simulink model "Areodynamic_Coefficient"  (R2022a)
settings: Solver=VariableStepAuto  StartTime=0.0  StopTime=1  RelTol=1e-3
undefined symbols (not defined in the file): a1, ac, AeroCoeff, b1
libraries: aerolibconvert2 x4
(part 1 of 2)
settings Model: Creator=user  LastModifiedBy=user
settings SolverCC: AlgebraicLoopSolver=TrustRegion
settings DataIOCC: SaveOutput=off  SaveTime=off  ReturnWorkspaceOutputs=off
settings DebuggingCC: UnconnectedInputMsg=warning  UnconnectedOutputMsg=warning  UnconnectedLineMsg=warning  SFMachineParentedDataDiag=warning

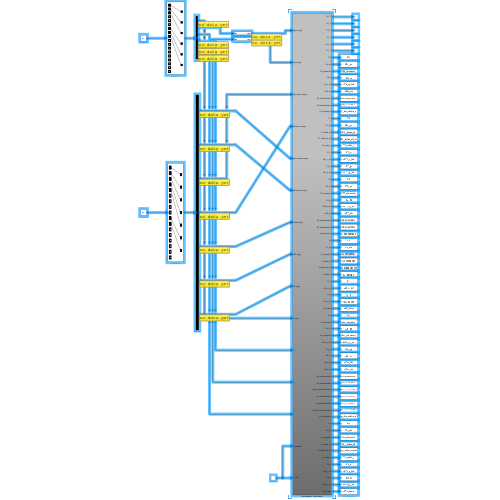
[thumbnail: Simulink's stored preview of the top-level diagram]
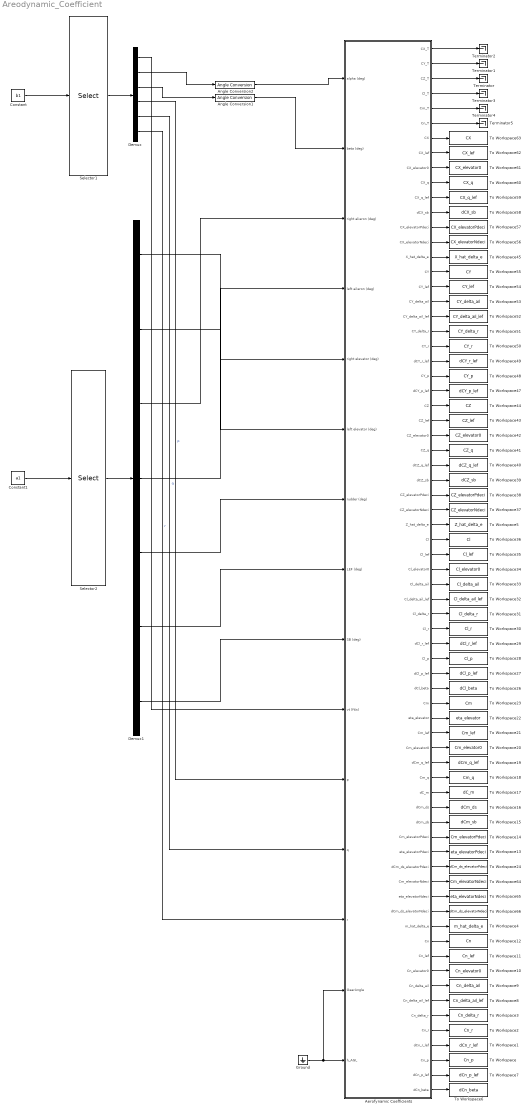
== system Areodynamic_Coefficient ==
  Aerofynamic Coefficients : Subsystem
  Angle Conversion1 : aerolibconvert2/Angle Conversion  IU=rad  OU=deg
  Angle Conversion2 : aerolibconvert2/Angle Conversion  IU=rad  OU=deg
  Constant : Constant  Value=b1
  Constant1 : Constant  Value=a1
  Demux : Demux  Outputs=6
  Demux1 : Demux  Outputs=7
  Ground : Ground
  Selector1 : Selector  InputPortWidth=18  IndexOptions=Index vector (dialog)  Indices=[1:3,7:9]  OutputSizes=3
  Selector2 : Selector  InputPortWidth=17  IndexOptions=Index vector (dialog)  Indices=[1:5 10 11]  OutputSizes=3
  Terminator{,1..5} (6 alike) : Terminator
  To Workspace : ToWorkspace  VariableName=Cn_p  SampleTime=-1
  To Workspace1 : ToWorkspace  VariableName=dCn_r_lef  SampleTime=-1
  To Workspace10 : ToWorkspace  VariableName=Cn_elevator0  SampleTime=-1
  To Workspace11 : ToWorkspace  VariableName=Cn_lef  SampleTime=-1
  To Workspace12 : ToWorkspace  VariableName=Cn  SampleTime=-1
  To Workspace13 : ToWorkspace  VariableName=eta_elevatorPdeci  SampleTime=-1
  To Workspace14 : ToWorkspace  VariableName=Cm_elevatorPdeci  SampleTime=-1
  To Workspace15 : ToWorkspace  VariableName=dCm_sb  SampleTime=-1
  To Workspace16 : ToWorkspace  VariableName=dCm_ds  SampleTime=-1
  To Workspace17 : ToWorkspace  VariableName=dC_m  SampleTime=-1
  To Workspace18 : ToWorkspace  VariableName=Cm_q  SampleTime=-1
  To Workspace19 : ToWorkspace  VariableName=dCm_q_lef  SampleTime=-1
  To Workspace2 : ToWorkspace  VariableName=Cn_r  SampleTime=-1
  To Workspace20 : ToWorkspace  VariableName=Cm_elevator0  SampleTime=-1
  To Workspace21 : ToWorkspace  VariableName=Cm_lef  SampleTime=-1
  To Workspace22 : ToWorkspace  VariableName=eta_elevator  SampleTime=-1
  To Workspace23 : ToWorkspace  VariableName=Cm  SampleTime=-1
  To Workspace24 : ToWorkspace  VariableName=dCm_ds_elevatorPdeci  SampleTime=-1
  To Workspace26 : ToWorkspace  VariableName=dCl_beta  SampleTime=-1
  To Workspace27 : ToWorkspace  VariableName=dCl_p_lef  SampleTime=-1
  To Workspace28 : ToWorkspace  VariableName=Cl_p  SampleTime=-1
  To Workspace29 : ToWorkspace  VariableName=dCl_r_lef  SampleTime=-1
  To Workspace3 : ToWorkspace  VariableName=Cn_delta_r  SampleTime=-1
  To Workspace30 : ToWorkspace  VariableName=Cl_r  SampleTime=-1
  To Workspace31 : ToWorkspace  VariableName=Cl_delta_r  SampleTime=-1
  To Workspace32 : ToWorkspace  VariableName=Cl_delta_ail_lef  SampleTime=-1
  To Workspace33 : ToWorkspace  VariableName=Cl_delta_ail  SampleTime=-1
  To Workspace34 : ToWorkspace  VariableName=Cl_elevator0  SampleTime=-1
  To Workspace35 : ToWorkspace  VariableName=Cl_lef  SampleTime=-1
  To Workspace36 : ToWorkspace  VariableName=Cl  SampleTime=-1
  To Workspace37 : ToWorkspace  VariableName=CZ_elevatorNdeci  SampleTime=-1
  To Workspace38 : ToWorkspace  VariableName=CZ_elevatorPdeci  SampleTime=-1
  To Workspace39 : ToWorkspace  VariableName=dCZ_sb  SampleTime=-1
  To Workspace4 : ToWorkspace  VariableName=m_hat_delta_e  SampleTime=-1
  To Workspace40 : ToWorkspace  VariableName=dCZ_q_lef  SampleTime=-1
  To Workspace41 : ToWorkspace  VariableName=CZ_q  SampleTime=-1
  To Workspace42 : ToWorkspace  VariableName=CZ_elevator0  SampleTime=-1
  To Workspace43 : ToWorkspace  VariableName=CZ_lef  SampleTime=-1
  To Workspace44 : ToWorkspace  VariableName=CZ  SampleTime=-1
  To Workspace45 : ToWorkspace  VariableName=X_hat_delta_e  SampleTime=-1
  To Workspace47 : ToWorkspace  VariableName=dCY_p_lef  SampleTime=-1
  To Workspace48 : ToWorkspace  VariableName=CY_p  SampleTime=-1
  To Workspace49 : ToWorkspace  VariableName=dCY_r_lef  SampleTime=-1
  To Workspace5 : ToWorkspace  VariableName=Z_hat_delta_e  SampleTime=-1
  To Workspace50 : ToWorkspace  VariableName=CY_r  SampleTime=-1
  To Workspace51 : ToWorkspace  VariableName=CY_delta_r  SampleTime=-1
  To Workspace52 : ToWorkspace  VariableName=CY_delta_ail_lef  SampleTime=-1
  To Workspace53 : ToWorkspace  VariableName=CY_delta_ail  SampleTime=-1
  To Workspace54 : ToWorkspace  VariableName=CY_lef  SampleTime=-1
  To Workspace55 : ToWorkspace  VariableName=CY  SampleTime=-1
  To Workspace56 : ToWorkspace  VariableName=CX_elevatorNdeci  SampleTime=-1
  To Workspace57 : ToWorkspace  VariableName=CX_elevatorPdeci  SampleTime=-1
  To Workspace58 : ToWorkspace  VariableName=dCX_sb  SampleTime=-1
  To Workspace59 : ToWorkspace  VariableName=CX_q_lef  SampleTime=-1
  To Workspace6 : ToWorkspace  VariableName=dCn_beta  SampleTime=-1
  To Workspace60 : ToWorkspace  VariableName=CX_q  SampleTime=-1
  To Workspace61 : ToWorkspace  VariableName=CX_elevator0  SampleTime=-1
  To Workspace62 : ToWorkspace  VariableName=CX_lef  SampleTime=-1
  To Workspace63 : ToWorkspace  VariableName=CX  SampleTime=-1
  To Workspace64 : ToWorkspace  VariableName=Cm_elevatorNdeci  SampleTime=-1
  To Workspace65 : ToWorkspace  VariableName=eta_elevatorNdeci  SampleTime=-1
  To Workspace66 : ToWorkspace  VariableName=dCm_ds_elevatorNdeci  SampleTime=-1
  To Workspace7 : ToWorkspace  VariableName=dCn_p_lef  SampleTime=-1
  To Workspace8 : ToWorkspace  VariableName=Cn_delta_ail_lef  SampleTime=-1
  To Workspace9 : ToWorkspace  VariableName=Cn_delta_ail  SampleTime=-1
  wires:
  Ground/1 -> Aerofynamic Coefficients/14(GearAngle), Aerofynamic Coefficients/15(h_AGL)
  Aerofynamic Coefficients/3(CZ_T) -> Terminator/1
  Aerofynamic Coefficients/2(CY_T) -> Terminator1/1
  Aerofynamic Coefficients/1(CX_T) -> Terminator2/1
  Aerofynamic Coefficients/4(Cl_T) -> Terminator3/1
  Aerofynamic Coefficients/5(Cm_T) -> Terminator4/1
  Aerofynamic Coefficients/6(Cn_T) -> Terminator5/1
  Aerofynamic Coefficients/69(Cn_p) -> To Workspace/1
  Angle Conversion1/1 -> Aerofynamic Coefficients/2(beta (deg))
  Angle Conversion2/1 -> Aerofynamic Coefficients/1(alpha (deg))
  Demux/2 -> Angle Conversion2/1
  Selector1/1 -> Demux/1
  Demux/3 -> Angle Conversion1/1
  Demux/1 -> Aerofynamic Coefficients/10(vt (ft/s))
  Constant1/1 -> Selector2/1
  Selector2/1 -> Demux1/1
  Demux1/1 -> Aerofynamic Coefficients/5(right elevator (deg))
  Demux1/2 -> Aerofynamic Coefficients/6(left elevator (deg))
  Demux1/3 -> Aerofynamic Coefficients/3(right alieron (deg))
  Demux1/4 -> Aerofynamic Coefficients/4(left aileron (deg))
  Demux1/5 -> Aerofynamic Coefficients/7(rudder (deg))
  Demux1/6 -> Aerofynamic Coefficients/8(LEF (deg))
  Demux1/7 -> Aerofynamic Coefficients/9(SB (deg))
  Aerofynamic Coefficients/68(dCn_r_lef) -> To Workspace1/1
  Aerofynamic Coefficients/67(Cn_r) -> To Workspace2/1
  Aerofynamic Coefficients/66(Cn_delta_r) -> To Workspace3/1
  Aerofynamic Coefficients/71(dCn_beta) -> To Workspace6/1
  Aerofynamic Coefficients/70(dCn_p_lef) -> To Workspace7/1
  Aerofynamic Coefficients/65(Cn_delta_ail_lef) -> To Workspace8/1
  Aerofynamic Coefficients/64(Cn_delta_ail) -> To Workspace9/1
  Aerofynamic Coefficients/63(Cn_elevator0) -> To Workspace10/1
  Aerofynamic Coefficients/62(Cn_lef) -> To Workspace11/1
  Aerofynamic Coefficients/61(Cn) -> To Workspace12/1
  Aerofynamic Coefficients/55(eta_elevatorPdeci) -> To Workspace13/1
  Aerofynamic Coefficients/54(Cm_elevatorPdeci) -> To Workspace14/1
  Aerofynamic Coefficients/53(dCm_sb) -> To Workspace15/1
  Aerofynamic Coefficients/52(dCm_ds) -> To Workspace16/1
  Aerofynamic Coefficients/51(dC_m) -> To Workspace17/1
  Aerofynamic Coefficients/50(Cm_q) -> To Workspace18/1
  Aerofynamic Coefficients/49(dCm_q_lef) -> To Workspace19/1
  Aerofynamic Coefficients/48(Cm_elevator0) -> To Workspace20/1
  Aerofynamic Coefficients/47(Cm_lef) -> To Workspace21/1
  Aerofynamic Coefficients/46(eta_elevator) -> To Workspace22/1
  Aerofynamic Coefficients/45(Cm) -> To Workspace23/1
  Aerofynamic Coefficients/44(dCl_beta) -> To Workspace26/1
  Aerofynamic Coefficients/43(dCl_p_lef) -> To Workspace27/1
  Aerofynamic Coefficients/42(Cl_p) -> To Workspace28/1
  Aerofynamic Coefficients/41(dCl_r_lef) -> To Workspace29/1
  Aerofynamic Coefficients/40(Cl_r) -> To Workspace30/1
  Aerofynamic Coefficients/39(Cl_delta_r) -> To Workspace31/1
  Aerofynamic Coefficients/38(Cl_delta_ail_lef) -> To Workspace32/1
  Aerofynamic Coefficients/37(Cl_delta_ail) -> To Workspace33/1
  Aerofynamic Coefficients/36(Cl_elevator0) -> To Workspace34/1
  Aerofynamic Coefficients/35(Cl_lef) -> To Workspace35/1
  Aerofynamic Coefficients/34(Cl) -> To Workspace36/1
  Aerofynamic Coefficients/32(CZ_elevatorNdeci) -> To Workspace37/1
  Aerofynamic Coefficients/31(CZ_elevatorPdeci) -> To Workspace38/1
  Aerofynamic Coefficients/30(dCZ_sb) -> To Workspace39/1
  Aerofynamic Coefficients/29(dCZ_q_lef) -> To Workspace40/1
  Aerofynamic Coefficients/28(CZ_q) -> To Workspace41/1
  Aerofynamic Coefficients/27(CZ_elevator0) -> To Workspace42/1
  Aerofynamic Coefficients/26(CZ_lef) -> To Workspace43/1
  Aerofynamic Coefficients/25(CZ) -> To Workspace44/1
  Aerofynamic Coefficients/24(dCY_p_lef) -> To Workspace47/1
  Aerofynamic Coefficients/23(CY_p) -> To Workspace48/1
  Aerofynamic Coefficients/22(dCY_r_lef) -> To Workspace49/1
  Aerofynamic Coefficients/21(CY_r) -> To Workspace50/1
  Aerofynamic Coefficients/20(CY_delta_r) -> To Workspace51/1
  Aerofynamic Coefficients/19(CY_delta_ail_lef) -> To Workspace52/1
  Aerofynamic Coefficients/18(CY_delta_ail) -> To Workspace53/1
  Aerofynamic Coefficients/17(CY_lef) -> To Workspace54/1
  Aerofynamic Coefficients/16(CY) -> To Workspace55/1
  Aerofynamic Coefficients/14(CX_elevatorNdeci) -> To Workspace56/1
  Aerofynamic Coefficients/13(CX_elevatorPdeci) -> To Workspace57/1
  Aerofynamic Coefficients/12(dCX_sb) -> To Workspace58/1
  Aerofynamic Coefficients/11(CX_q_lef) -> To Workspace59/1
  Aerofynamic Coefficients/10(CX_q) -> To Workspace60/1
  Aerofynamic Coefficients/9(CX_elevator0) -> To Workspace61/1
  Aerofynamic Coefficients/8(CX_lef) -> To Workspace62/1
  Aerofynamic Coefficients/7(CX) -> To Workspace63/1
  Aerofynamic Coefficients/56(dCm_ds_elevatorPdeci) -> To Workspace24/1
  Aerofynamic Coefficients/57(Cm_elevatorNdeci) -> To Workspace64/1
  Aerofynamic Coefficients/58(eta_elevatorNdeci) -> To Workspace65/1
  Aerofynamic Coefficients/59(dCm_ds_elevatorNdeci) -> To Workspace66/1
  Aerofynamic Coefficients/60(m_hat_delta_e) -> To Workspace4/1
  Aerofynamic Coefficients/33(Z_hat_delta_e) -> To Workspace5/1
  Aerofynamic Coefficients/15(X_hat_delta_e) -> To Workspace45/1
  Constant/1 -> Selector1/1
  Demux/6 -> Aerofynamic Coefficients/13(r)  "r"
  Demux/5 -> Aerofynamic Coefficients/12(q)  "q"
  Demux/4 -> Aerofynamic Coefficients/11(p)  "p"

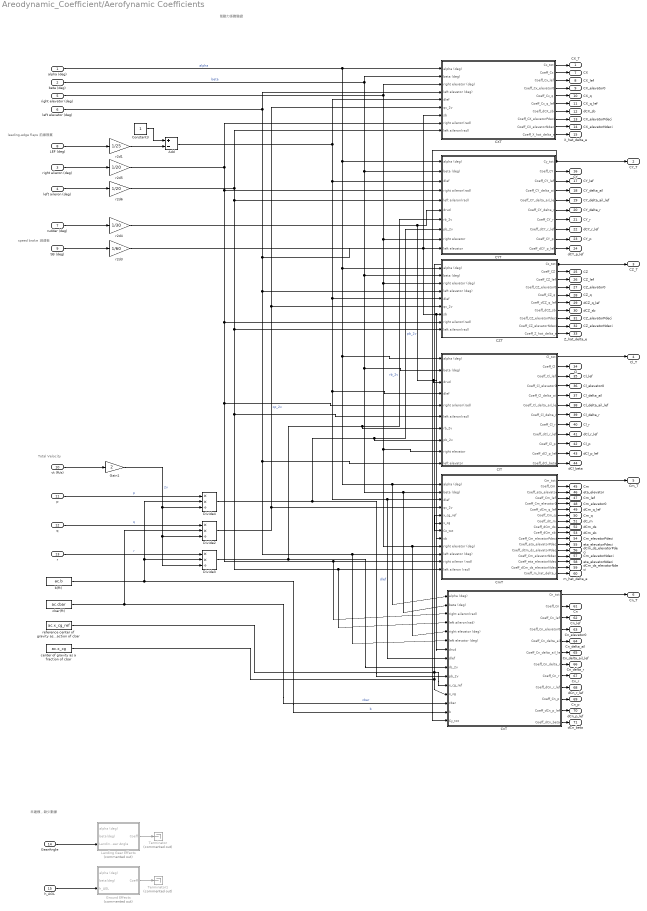
== system Areodynamic_Coefficient/Aerofynamic Coefficients ==
  note: 氣動力係數驗證
  note: Total Velocity
  note: 未建模，缺少數據
  note: speed brake
      | 減速板
  note: leading-edge flaps
      | 前緣襟翼
  alpha (deg) : Inport
  beta (deg) : Inport  Port=2
  right alieron (deg) : Inport  Port=3
  left aileron (deg) : Inport  Port=4
  right elevator (deg) : Inport  Port=5
  left elevator (deg) : Inport  Port=6
  rudder (deg) : Inport  Port=7
  LEF (deg) : Inport  Port=8
  SB (deg) : Inport  Port=9
  vt (ft/s) : Inport  Port=10
  p : Inport  Port=11
  q : Inport  Port=12
  r : Inport  Port=13
  GearAngle : Inport  Port=14
  h_AGL : Inport  Port=15
  Add : Sum  Inputs=+-
  CXT : Subsystem
  CYT : Subsystem
  CZT : Subsystem
  ClT : Subsystem
  CmT : Subsystem
  CnT : Subsystem
  Constant3 : Constant
  Divide2 : Product  Inputs=**/
  Divide3 : Product  Inputs=**/
  Divide4 : Product  Inputs=**/
  Gain1 : Gain  Gain=2
  Ground Effects : Subsystem  Commented=on
  Landing Gear Effects : Subsystem  Commented=on
  Terminator : Terminator  Commented=on
  Terminator1 : Terminator  Commented=on
  b(ft) : Constant  Value=ac.b
  cbar(ft) : Constant  Value=ac.cbar
  center of gravity as a fraction of cbar : Constant  Value=ac.x_cg
  r2d1 : Gain  Gain=1/25  SaturateOnIntegerOverflow=on  OutDataTypeStr=Inherit: Same as input  ParamDataTypeStr=Inherit: Same as input
  r2d3 : Gain  Gain=1/60  SaturateOnIntegerOverflow=on  OutDataTypeStr=Inherit: Same as input  ParamDataTypeStr=Inherit: Same as input
  r2d4 : Gain  Gain=1/30  SaturateOnIntegerOverflow=on  OutDataTypeStr=Inherit: Same as input  ParamDataTypeStr=Inherit: Same as input
  r2d5 : Gain  Gain=1/20  SaturateOnIntegerOverflow=on  OutDataTypeStr=Inherit: Same as input  ParamDataTypeStr=Inherit: Same as input
  r2d6 : Gain  Gain=1/20  SaturateOnIntegerOverflow=on  OutDataTypeStr=Inherit: Same as input  ParamDataTypeStr=Inherit: Same as input
  reference center of gravity as a fraction of cbar : Constant  Value=ac.x_cg_ref
  CX_T : Outport  VectorParamsAs1DForOutWhenUnconnected=off
  CY_T : Outport  Port=2  VectorParamsAs1DForOutWhenUnconnected=off
  CZ_T : Outport  Port=3  VectorParamsAs1DForOutWhenUnconnected=off
  Cl_T : Outport  Port=4  VectorParamsAs1DForOutWhenUnconnected=off
  Cm_T : Outport  Port=5  VectorParamsAs1DForOutWhenUnconnected=off
  Cn_T : Outport  Port=6  VectorParamsAs1DForOutWhenUnconnected=off
  CX : Outport  Port=7  VectorParamsAs1DForOutWhenUnconnected=off
  CX_lef : Outport  Port=8  VectorParamsAs1DForOutWhenUnconnected=off
  CX_elevator0 : Outport  Port=9  VectorParamsAs1DForOutWhenUnconnected=off
  CX_q : Outport  Port=10  VectorParamsAs1DForOutWhenUnconnected=off
  CX_q_lef : Outport  Port=11  VectorParamsAs1DForOutWhenUnconnected=off
  dCX_sb : Outport  Port=12  VectorParamsAs1DForOutWhenUnconnected=off
  CX_elevatorPdeci : Outport  Port=13  VectorParamsAs1DForOutWhenUnconnected=off
  CX_elevatorNdeci : Outport  Port=14  VectorParamsAs1DForOutWhenUnconnected=off
  X_hat_delta_e : Outport  Port=15
  CY : Outport  Port=16
  CY_lef : Outport  Port=17
  CY_delta_ail : Outport  Port=18
  CY_delta_ail_lef : Outport  Port=19
  CY_delta_r : Outport  Port=20
  CY_r : Outport  Port=21
  dCY_r_lef : Outport  Port=22
  CY_p : Outport  Port=23
  dCY_p_lef : Outport  Port=24
  CZ : Outport  Port=25
  CZ_lef : Outport  Port=26
  CZ_elevator0 : Outport  Port=27
  CZ_q : Outport  Port=28
  dCZ_q_lef : Outport  Port=29
  dCZ_sb : Outport  Port=30
  CZ_elevatorPdeci : Outport  Port=31
  CZ_elevatorNdeci : Outport  Port=32
  Z_hat_delta_e : Outport  Port=33
  Cl : Outport  Port=34
  Cl_lef : Outport  Port=35
  Cl_elevator0 : Outport  Port=36
  Cl_delta_ail : Outport  Port=37
  Cl_delta_ail_lef : Outport  Port=38
  Cl_delta_r : Outport  Port=39
  Cl_r : Outport  Port=40
  dCl_r_lef : Outport  Port=41
  Cl_p : Outport  Port=42
  dCl_p_lef : Outport  Port=43
  dCl_beta : Outport  Port=44
  Cm : Outport  Port=45
  eta_elevator : Outport  Port=46
  Cm_lef : Outport  Port=47
  Cm_elevator0 : Outport  Port=48
  dCm_q_lef : Outport  Port=49
  Cm_q : Outport  Port=50
  dC_m : Outport  Port=51
  dCm_ds : Outport  Port=52
  dCm_sb : Outport  Port=53
  Cm_elevatorPdeci : Outport  Port=54
  eta_elevatorPdeci : Outport  Port=55
  dCm_ds_elevatorPdeci : Outport  Port=56
  Cm_elevatorNdeci : Outport  Port=57
  eta_elevatorNdeci : Outport  Port=58
  dCm_ds_elevatorNdeci : Outport  Port=59
  m_hat_delta_e : Outport  Port=60
  Cn : Outport  Port=61
  Cn_lef : Outport  Port=62
  Cn_elevator0 : Outport  Port=63
  Cn_delta_ail : Outport  Port=64
  Cn_delta_ail_lef : Outport  Port=65
  Cn_delta_r : Outport  Port=66
  Cn_r : Outport  Port=67
  dCn_r_lef : Outport  Port=68
  Cn_p : Outport  Port=69
  dCn_p_lef : Outport  Port=70
  dCn_beta : Outport  Port=71
  wires:
  alpha (deg)/1 -> CnT/1(alpha (deg)), CmT/1(alpha (deg)), ClT/1(alpha (deg)), CZT/1(alpha (deg)), CYT/1(alpha (deg)), CXT/1(alpha (deg))  "alpha"
  beta (deg)/1 -> CnT/2(beta (deg)), CmT/2(beta (deg)), ClT/2(beta (deg)), CZT/2(beta (deg)), CYT/2(beta (deg)), CXT/2("beta (deg) ")  "beta"
  right elevator (deg)/1 -> CnT/5("right elevator (deg) "), CmT/9(right elevator (deg)), ClT/9(right elevator), CZT/3(right elevator (deg)), CYT/9(right elevator), CXT/3(right elevator (deg))
  vt (ft/s)/1 -> Gain1/1
  q/1 -> Divide2/1  "q"
  r/1 -> Divide3/1  "r"
  Divide2/1 -> CXT/6(qc_2v), CZT/6(qc_2v), CmT/4(qc_2v)  "qc_2v"
  Divide3/1 -> CYT/7(rb_2v), ClT/7(rb_2v), CnT/9(rb_2v)  "rb_2v"
  Divide4/1 -> CYT/8(pb_2v), ClT/8(pb_2v), CnT/10(pb_2v)  "pb_2v"
  b(ft)/1 -> CnT/14(b), Divide3/2, Divide4/2  "b"
  cbar(ft)/1 -> CnT/13(cbar), Divide2/2  "cbar"
  reference center of gravity as a fraction of cbar/1 -> CmT/5(x_cg_ref), CnT/11(x_cg_ref)
  center of gravity as a fraction of cbar/1 -> CmT/6(x_cg), CnT/12(x_cg)
  CZT/1(Cz_tot) -> CZ_T/1, CmT/7(Cz_tot)
  CYT/1(Cy_tot) -> CY_T/1, CnT/15(Cy_tot)
  CXT/1(Cx_tot) -> CX_T/1
  ClT/1(Cl_tot) -> Cl_T/1
  CmT/1(Cm_tot) -> Cm_T/1
  CnT/1(Cn_tot) -> Cn_T/1
  Add/1 -> CXT/5(dlef), CnT/8(dlef), CmT/3(dlef), ClT/4(dlef), CZT/5(dlef), CYT/3(dlef)  "dlef"
  rudder (deg)/1 -> r2d4/1
  SB (deg)/1 -> r2d3/1
  r2d1/1 -> Add/2
  Constant3/1 -> Add/1
  LEF (deg)/1 -> r2d1/1
  Gain1/1 -> Divide4/3, Divide3/3, Divide2/3  "2v"
  p/1 -> Divide4/1  "p"
  r2d3/1 -> CmT/8(sb), CZT/7(sb), CXT/7(sb)
  r2d4/1 -> CYT/6(drud), CnT/7(drud), ClT/3(drud)
  GearAngle/1 -> Landing Gear Effects/3(Landing Gear Angle)
  h_AGL/1 -> Ground Effects/3(h_AGL)
  Landing Gear Effects/1(Coeff) -> Terminator/1
  Ground Effects/1(Coeff) -> Terminator1/1
  left elevator (deg)/1 -> CnT/6(left elevator (deg)), CmT/10(left elevator (deg)), ClT/10(left elevator), CZT/4(left elevator (deg)), CYT/10(left elevator), CXT/4(left elevator (deg))
  right alieron (deg)/1 -> r2d5/1
  left aileron (deg)/1 -> r2d6/1
  r2d5/1 -> CnT/3(right aileron(rad)), CmT/11(right aileron (rad)), ClT/5(right aileron(rad)), CZT/8(right aileron(rad)), CYT/4(right aileron(rad)), CXT/8(right aileron(rad))
  r2d6/1 -> CXT/9(left aileron(rad)), CnT/4(left aileron(rad)), CmT/12(left aileron (rad)), ClT/6(left aileron(rad)), CZT/9(left aileron(rad)), CYT/5(left aileron(rad))
  CnT/10(Coeff_Cn_p) -> Cn_p/1
  CXT/2(Coeff_Cx) -> CX/1
  CXT/3(Coeff_Cx_lef) -> CX_lef/1
  CXT/4(Coeff_Cx_elevator0) -> CX_elevator0/1
  CXT/5(Coeff_Cx_q) -> CX_q/1
  CXT/6(Coeff_Cx_q_lef) -> CX_q_lef/1
  CXT/7(Coeff_dCX_sb) -> dCX_sb/1
  CXT/8(Coeff_CX_elevatorPdeci) -> CX_elevatorPdeci/1
  CXT/9(Coeff_CX_elevatorNdeci) -> CX_elevatorNdeci/1
  CYT/2(Coeff_CY) -> CY/1
  CYT/3(Coeff_CY_lef) -> CY_lef/1
  CYT/4(Coeff_CY_delta_ail) -> CY_delta_ail/1
  CYT/5(Coeff_CY_delta_ail_lef) -> CY_delta_ail_lef/1
  CYT/6(Coeff_CY_delta_r) -> CY_delta_r/1
  CYT/7(Coeff_CY_r) -> CY_r/1
  CYT/8(Coeff_dCY_r_lef) -> dCY_r_lef/1
  CYT/9(Coeff_CY_p) -> CY_p/1
  CYT/10(Coeff_dCY_p_lef) -> dCY_p_lef/1
  CZT/2(Coeff_CZ) -> CZ/1
  CZT/3(Coeff_CZ_lef) -> CZ_lef/1
  CZT/4(Coeff_CZ_elevator0) -> CZ_elevator0/1
  CZT/5(Coeff_CZ_q) -> CZ_q/1
  CZT/6(Coeff_dCZ_q_lef) -> dCZ_q_lef/1
  CZT/7(Coeff_dCZ_sb) -> dCZ_sb/1
  CZT/8(Coeff_CZ_elevatorPdeci) -> CZ_elevatorPdeci/1
  CZT/9(Coeff_CZ_elevatorNdeci) -> CZ_elevatorNdeci/1
  ClT/2(Coeff_Cl) -> Cl/1
  ClT/3(Coeff_Cl_lef) -> Cl_lef/1
  ClT/4(Coeff_Cl_elevator0) -> Cl_elevator0/1
  ClT/5(Coeff_Cl_delta_ail) -> Cl_delta_ail/1
  ClT/6(Coeff_Cl_delta_ail_lef) -> Cl_delta_ail_lef/1
  ClT/7(Coeff_Cl_delta_r) -> Cl_delta_r/1
  ClT/8(Coeff_Cl_r) -> Cl_r/1
  ClT/9(Coeff_dCl_r_lef) -> dCl_r_lef/1
  ClT/10(Coeff_Cl_p) -> Cl_p/1
  ClT/11(Coeff_dCl_p_lef) -> dCl_p_lef/1
  ClT/12(Coeff_dCl_beta) -> dCl_beta/1
  CmT/2(Coeff_Cm) -> Cm/1
  CmT/3(Coeff_eta_elevator) -> eta_elevator/1
  CmT/4(Coeff_Cm_lef) -> Cm_lef/1
  CmT/5(Coeff_Cm_elevator0) -> Cm_elevator0/1
  CmT/6(Coeff_dCm_q_lef) -> dCm_q_lef/1
  CmT/7(Coeff_Cm_q) -> Cm_q/1
  CmT/8(Coeff_dC_m) -> dC_m/1
  CmT/9(Coeff_dCm_ds) -> dCm_ds/1
  CmT/10(Coeff_dCm_sb) -> dCm_sb/1
  CmT/11(Coeff_Cm_elevatorPdeci) -> Cm_elevatorPdeci/1
  CmT/12(Coeff_eta_elevatorPdeci) -> eta_elevatorPdeci/1
  CnT/3(Coeff_Cn_lef) -> Cn_lef/1
  CnT/2(Coeff_Cn) -> Cn/1
  CnT/4(Coeff_Cn_elevator0) -> Cn_elevator0/1
  CnT/5(Coeff_Cn_delta_ail) -> Cn_delta_ail/1
  CnT/6(Coeff_Cn_delta_ail_lef) -> Cn_delta_ail_lef/1
  CnT/7(Coeff_Cn_delta_r) -> Cn_delta_r/1
  CnT/8(Coeff_Cn_r) -> Cn_r/1
  CnT/9(Coeff_dCn_r_lef) -> dCn_r_lef/1
  CnT/11(Coeff_dCn_p_lef) -> dCn_p_lef/1
  CnT/12(Coeff_dCn_beta) -> dCn_beta/1
  CmT/13(Coeff_dCm_ds_elevatorPdeci) -> dCm_ds_elevatorPdeci/1
  CmT/14(Coeff_Cm_elevatorNdeci) -> Cm_elevatorNdeci/1
  CmT/15(Coeff_eta_elevatorNdeci) -> eta_elevatorNdeci/1
  CmT/16(Coeff_dCm_ds_elevatorNdeci) -> dCm_ds_elevatorNdeci/1
  CXT/10(Coeff_X_hat_delta_e) -> X_hat_delta_e/1
  CZT/10(Coeff_Z_hat_delta_e) -> Z_hat_delta_e/1
  CmT/17(Coeff_m_hat_delta_e) -> m_hat_delta_e/1

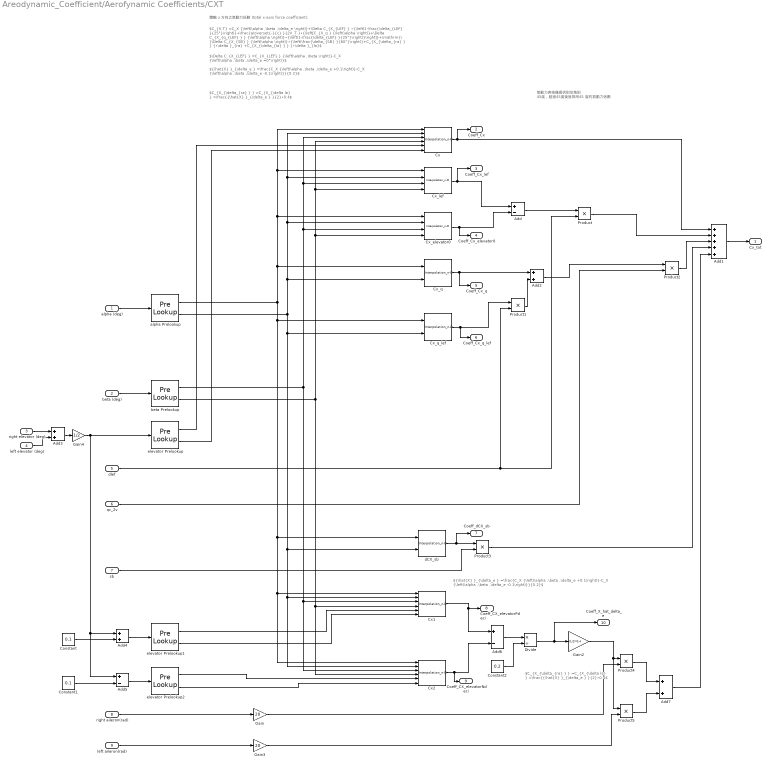
== system Areodynamic_Coefficient/Aerofynamic Coefficients/CXT ==
  note: 氣動力表格僅提供到攻角到
      | 45度，超過45度後皆採用45
      | 度的氣動力係數
  note: $C_{X,T} =C_X {\left(\alpha ,\beta ,\delta_e \right)}+\Delta C_{X_{LEF} } ∙{\left(1-\frac{\delta_{LEF} }{25°}\right)}+\frac{q\overset{-}{c} }{2V_T }∙{\left[C_{X_q } {\left(\alpha \right)}+\Delta C_{X_{q_{LEF} } } {\left(\alpha \right)}∙{\left(1-\frac{\delta_{LEF} }{25°}\right)}\right]}+\mathrm{\ }\Delta C_{X_{SB} } {\left(\alpha \right)}∙{\left(\frac{\delta_{SB} }{60°}\right)}+C_{X_{\delta_{ra} } } {∙\delta }_{ra} +C_{X_{\delta_{la} } } {∙\delta }_{la}$
  note: 體軸 x 方向之氣動力係數 (total x-axis force coefficient)：
  note: ${\hat{X} }_{\delta_e } =\frac{C_X {\left(\alpha ,\beta ,\delta_e +0.1\right)}-C_X {\left(\alpha ,\beta ,\delta_e -0.1\right)}}{0.2}$
  note: $C_{X_{\delta_{ra} } } =C_{X_{\delta la} } =\frac{{\hat{X} }_{\delta_e } }{2}∙0.4$
  note: $\Delta C_{X_{LEF} } =C_{X_{LEF} } {\left(\alpha ,\beta \right)}-C_X {\left(\alpha ,\beta ,\delta_e =0°\right)}$
  note: ${\hat{X} }_{\delta_e } =\frac{C_X {\left(\alpha ,\beta ,\delta_e +0.1\right)}-C_X {\left(\alpha ,\beta ,\delta_e -0.1\right)}}{0.2}$
  note: $C_{X_{\delta_{ra} } } =C_{X_{\delta la} } =\frac{{\hat{X} }_{\delta_e } }{2}∙0.4$
  alpha (deg) : Inport
  "beta (deg) " : Inport  Port=2
  right elevator (deg) : Inport  Port=3
  left elevator (deg) : Inport  Port=4
  dlef : Inport  Port=5
  qc_2v : Inport  Port=6
  sb : Inport  Port=7
  right aileron(rad) : Inport  Port=8
  left aileron(rad) : Inport  Port=9
  Add : Sum  Inputs=+-
  Add1 : Sum  Inputs=+++++
  Add{2..4,7} (4 alike) : Sum
  Add5 : Sum  Inputs=+-
  Add6 : Sum  Inputs=+-
  Constant : Constant  Value=0.1
  Constant1 : Constant  Value=0.1
  Constant2 : Constant  Value=0.2
  Cx : Interpolation_n-D  NumberOfTableDimensions=3  Table=AeroCoeff.Cx
      settings: InputPortMap=u0,u1,u2,u3,u4,u5
  Cx1 : Interpolation_n-D  NumberOfTableDimensions=3  Table=AeroCoeff.Cx
      settings: InputPortMap=u0,u1,u2,u3,u4,u5
  Cx2 : Interpolation_n-D  NumberOfTableDimensions=3  Table=AeroCoeff.Cx
      settings: InputPortMap=u0,u1,u2,u3,u4,u5
  Cx_elevator0 : Interpolation_n-D  Table=AeroCoeff.Cx_elevator0
  Cx_lef : Interpolation_n-D  Table=AeroCoeff.Cx_lef
  "Cx_q " : Interpolation_n-D  NumberOfTableDimensions=1  Table=AeroCoeff.Cx_q
      settings: InputPortMap=u0,u1
  Cx_q_lef : Interpolation_n-D  NumberOfTableDimensions=1  Table=AeroCoeff.Cx_q_lef
      settings: InputPortMap=u0,u1
  Divide : Product  Inputs=*/
  Gain : Gain  Gain=20
  Gain2 : Gain  Gain=(1/2)*0.4
  Gain3 : Gain  Gain=20
  Gain4 : Gain  Gain=1/2
  Product{,1..5} (6 alike) : Product
  alpha Prelookup : PreLookup  BreakpointsData=AeroCoeff.alpha_prelookup  IndexSearchMethod=Linear search  BeginIndexSearchUsingPreviousIndexResult=on  DiagnosticForOutOfRangeInput=Warning
  beta Prelookup : PreLookup  BreakpointsData=AeroCoeff.beta_prelookup  IndexSearchMethod=Linear search  BeginIndexSearchUsingPreviousIndexResult=on  DiagnosticForOutOfRangeInput=Warning
  dCX_sb : Interpolation_n-D  NumberOfTableDimensions=1  Table=AeroCoeff.dCX_sb
      settings: InputPortMap=u0,u1
  elevator Prelookup : PreLookup  BreakpointsData=AeroCoeff.elevator_prelookup2  IndexSearchMethod=Linear search  BeginIndexSearchUsingPreviousIndexResult=on  DiagnosticForOutOfRangeInput=Warning
  elevator Prelookup1 : PreLookup  BreakpointsData=AeroCoeff.elevator_prelookup2  IndexSearchMethod=Linear search  BeginIndexSearchUsingPreviousIndexResult=on  DiagnosticForOutOfRangeInput=Warning
  elevator Prelookup2 : PreLookup  BreakpointsData=AeroCoeff.elevator_prelookup2  IndexSearchMethod=Linear search  BeginIndexSearchUsingPreviousIndexResult=on  DiagnosticForOutOfRangeInput=Warning
  Cx_tot : Outport  VectorParamsAs1DForOutWhenUnconnected=off
  Coeff_Cx : Outport  Port=2
  Coeff_Cx_lef : Outport  Port=3
  Coeff_Cx_elevator0 : Outport  Port=4
  Coeff_Cx_q : Outport  Port=5
  Coeff_Cx_q_lef : Outport  Port=6
  Coeff_dCX_sb : Outport  Port=7
  Coeff_CX_elevatorPdeci : Outport  Port=8
  Coeff_CX_elevatorNdeci : Outport  Port=9
  Coeff_X_hat_delta_e : Outport  Port=10
  wires:
  beta Prelookup/2 -> Cx2/4, Cx1/4, Cx_elevator0/4, Cx_lef/4, Cx/4
  beta Prelookup/1 -> Cx2/3, Cx1/3, Cx_elevator0/3, Cx_lef/3, Cx/3
  Cx_lef/1 -> Add/1, Coeff_Cx_lef/1
  alpha Prelookup/1 -> Cx_q_lef/1, Cx2/1, Cx1/1, dCX_sb/1, "Cx_q "/1, Cx_elevator0/1, Cx/1, Cx_lef/1
  elevator Prelookup/2 -> Cx/6
  "beta (deg) "/1 -> beta Prelookup/1
  Add/1 -> Product/1
  alpha Prelookup/2 -> Cx_q_lef/2, Cx2/2, Cx1/2, dCX_sb/2, "Cx_q "/2, Cx_elevator0/2, Cx_lef/2, Cx/2
  Product/1 -> Add1/2
  elevator Prelookup/1 -> Cx/5
  Add2/1 -> Product2/1
  Cx/1 -> Add1/1, Coeff_Cx/1
  Cx_elevator0/1 -> Coeff_Cx_elevator0/1, Add/2
  Cx_q_lef/1 -> Coeff_Cx_q_lef/1, Product1/1
  Product1/1 -> Add2/2
  "Cx_q "/1 -> Coeff_Cx_q/1, Add2/1
  dlef/1 -> Product/2, Product1/2
  Product2/1 -> Add1/3
  Add1/1 -> Cx_tot/1
  qc_2v/1 -> Product2/2
  dCX_sb/1 -> Coeff_dCX_sb/1, Product3/1
  sb/1 -> Product3/2
  Product3/1 -> Add1/4
  alpha (deg)/1 -> alpha Prelookup/1
  Add3/1 -> Gain4/1
  right elevator (deg)/1 -> Add3/1
  left elevator (deg)/1 -> Add3/2
  Add4/1 -> elevator Prelookup1/1
  Constant/1 -> Add4/2
  Constant1/1 -> Add5/2
  Add5/1 -> elevator Prelookup2/1
  elevator Prelookup1/1 -> Cx1/5
  elevator Prelookup1/2 -> Cx1/6
  Cx2/1 -> Coeff_CX_elevatorNdeci/1, Add6/2
  Add6/1 -> Divide/1
  Divide/1 -> Coeff_X_hat_delta_e/1, Gain2/1
  right aileron(rad)/1 -> Gain/1
  Gain2/1 -> Product5/1, Product4/1
  left aileron(rad)/1 -> Gain3/1
  Product4/1 -> Add7/1
  Product5/1 -> Add7/2
  Add7/1 -> Add1/5
  Constant2/1 -> Divide/2
  Gain/1 -> Product4/2
  Gain3/1 -> Product5/2
  elevator Prelookup2/1 -> Cx2/5
  elevator Prelookup2/2 -> Cx2/6
  Gain4/1 -> Add4/1, Add5/1, elevator Prelookup/1
  Cx1/1 -> Coeff_CX_elevatorPdeci/1, Add6/1

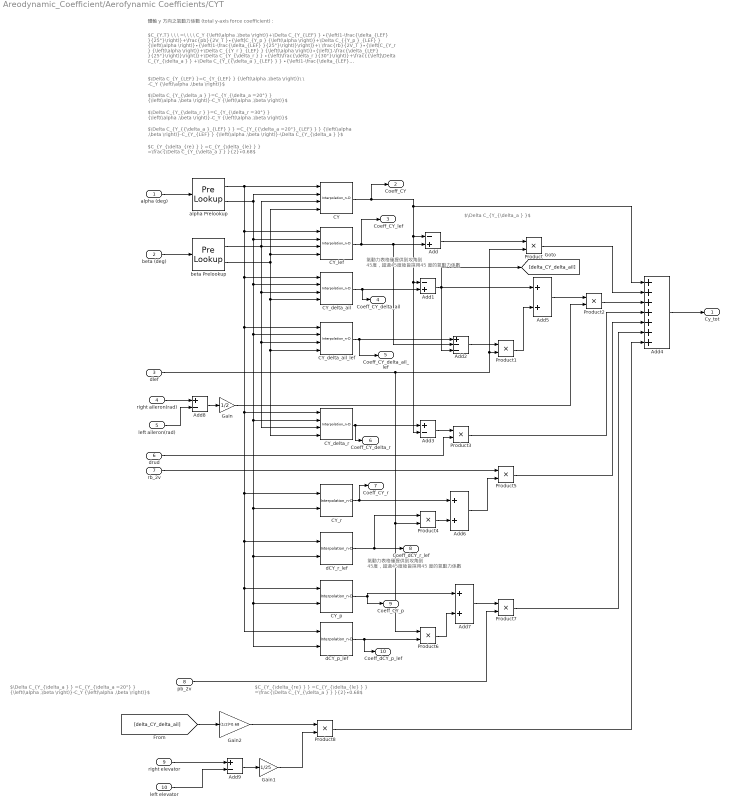
== system Areodynamic_Coefficient/Aerofynamic Coefficients/CYT ==
  note: $\Delta C_{Y_{\delta_a } }$
  note: 氣動力表格僅提供到攻角到
      | 45度，超過45度後皆採用45
      | 度的氣動力係數
  note: 氣動力表格僅提供到攻角到
      | 45度，超過45度後皆採用45
      | 度的氣動力係數
  note: 體軸 y 方向之氣動力係數 (total y-axis force coefficient)：
  note: $C_{Y_{\delta_{re} } } =C_{Y_{\delta_{le} } } =\frac{\Delta C_{Y_{\delta_a } } }{2}∙0.68$
  note: $C_{Y,T} \ \ \ =\ \ \ \ C_Y {\left(\alpha ,\beta \right)}+\Delta C_{Y_{LEF} } ∙{\left(1-\frac{\delta_{LEF} }{25°}\right)}+\frac{pb}{2V_T }∙{\left[C_{Y_p } {\left(\alpha \right)}+\Delta C_{{Y_p }_{LEF} } {\left(\alpha \right)}∙{\left(1-\frac{\delta_{LEF} }{25°}\right)}\right]}+\ \frac{rb}{2V_T }∙{\left[C_{Y_r } {\left(\alpha \right)}+\Delta C_{{Y_r }_{LEF} } {\left(\alpha \right)}∙{\left(1-\frac{\delta_{LEF} }{25°}\right)}\right]}+\Delta C_{Y_{\delta_r } } ∙{\left(\frac{\delta_r }{30°}\right)}+\frac{{\left[\Delta C_{Y_{\delta_a } } +\Delta C_{Y_{{\delta_a }_{LEF} } } ∙{\left(1-\frac{\delta_{LEF} }{25°}\right)}\right]}}{2}∙{\left(\frac{\delta_{ra} }{20°}\right)}-\frac{{\left[\Delta C_{Y_{\delta_a } } +\Delta C_{Y_{{\delta_a }_{LEF} } } ∙{\left(1-\frac{\delta_{LEF} }{25°}\right)}\right]}}{2}∙{\left(\frac{\delta_{la} }{20°}\right)}{+C}_{Y_{\delta_{re} } } ∙{\left(\frac{\delta_{re} }{25°}\right)}-C_{Y_{\delta_{le} } } ∙{\left(\frac{\delta_{le} }{25°}\right)}$
  note: $\Delta C_{Y_{\delta_r } }=C_{Y_{\delta_r =30°} } {\left(\alpha ,\beta \right)}-C_Y {\left(\alpha ,\beta \right)}$
  note: $\Delta C_{Y_{{\delta_a }_{LEF} } } =C_{Y_{{\delta_a =20°}_{LEF} } } {\left(\alpha ,\beta \right)}-C_{Y_{LEF} } {\left(\alpha ,\beta \right)}-\Delta C_{Y_{\delta_a } }$
  note: $\Delta C_{Y_{LEF} }=C_{Y_{LEF} } {\left(\alpha ,\beta \right)}\ \ -C_Y {\left(\alpha ,\beta \right)}$
  note: $\Delta C_{Y_{\delta_a } }=C_{Y_{\delta_a =20°} } {\left(\alpha ,\beta \right)}-C_Y {\left(\alpha ,\beta \right)}$
  note: $C_{Y_{\delta_{re} } } =C_{Y_{\delta_{le} } } =\frac{\Delta C_{Y_{\delta_a } } }{2}∙0.68$
  note: $\Delta C_{Y_{\delta_a } } =C_{Y_{\delta_a =20°} } {\left(\alpha ,\beta \right)}-C_Y {\left(\alpha ,\beta \right)}$
  alpha (deg) : Inport
  beta (deg) : Inport  Port=2
  dlef : Inport  Port=3
  right aileron(rad) : Inport  Port=4
  left aileron(rad) : Inport  Port=5
  drud : Inport  Port=6
  rb_2v : Inport  Port=7
  pb_2v : Inport  Port=8
  right elevator : Inport  Port=9
  left elevator : Inport  Port=10
  Add : Sum  Inputs=-+
  Add1 : Sum  Inputs=-+
  Add2 : Sum  Inputs=+--
  Add3 : Sum  Inputs=+-
  Add4 : Sum  Inputs=+++++++
  Add5 : Sum
  Add6 : Sum
  Add7 : Sum
  Add8 : Sum  Inputs=+-
  Add9 : Sum  Inputs=+-
  CY : Interpolation_n-D  Table=AeroCoeff.CY
  CY_delta_ail : Interpolation_n-D  Table=AeroCoeff.CY_delta_ail
  CY_delta_ail_lef : Interpolation_n-D  Table=AeroCoeff.CY_delta_ail_lef
  CY_delta_r : Interpolation_n-D  Table=AeroCoeff.CY_delta_r
  CY_lef : Interpolation_n-D  Table=AeroCoeff.CY_lef
  CY_p : Interpolation_n-D  NumberOfTableDimensions=1  Table=AeroCoeff.CY_p
      settings: InputPortMap=u0,u1
  CY_r : Interpolation_n-D  NumberOfTableDimensions=1  Table=AeroCoeff.CY_r
      settings: InputPortMap=u0,u1
  Gain : Gain  Gain=1/2
  Gain1 : Gain  Gain=1/25
  Gain2 : Gain  Gain=(1/2)*0.68
  Product{,1..8} (9 alike) : Product
  alpha Prelookup : PreLookup  BreakpointsData=AeroCoeff.alpha_prelookup  IndexSearchMethod=Linear search  BeginIndexSearchUsingPreviousIndexResult=on  DiagnosticForOutOfRangeInput=Warning
  beta Prelookup : PreLookup  BreakpointsData=AeroCoeff.beta_prelookup  IndexSearchMethod=Linear search  BeginIndexSearchUsingPreviousIndexResult=on  DiagnosticForOutOfRangeInput=Warning
  dCY_p_lef : Interpolation_n-D  NumberOfTableDimensions=1  Table=AeroCoeff.dCY_p_lef
      settings: InputPortMap=u0,u1
  dCY_r_lef : Interpolation_n-D  NumberOfTableDimensions=1  Table=AeroCoeff.dCY_r_lef
      settings: InputPortMap=u0,u1
  Cy_tot : Outport  VectorParamsAs1DForOutWhenUnconnected=off
  Coeff_CY : Outport  Port=2
  Coeff_CY_lef : Outport  Port=3
  Coeff_CY_delta_ail : Outport  Port=4
  Coeff_CY_delta_ail_lef : Outport  Port=5
  Coeff_CY_delta_r : Outport  Port=6
  Coeff_CY_r : Outport  Port=7
  Coeff_dCY_r_lef : Outport  Port=8
  Coeff_CY_p : Outport  Port=9
  Coeff_dCY_p_lef : Outport  Port=10
  wires:
  Add3/1 -> Product3/1
  beta Prelookup/2 -> CY_delta_r/4, CY_delta_ail_lef/4, CY_delta_ail/4, CY_lef/4, CY/4
  beta Prelookup/1 -> CY_lef/3, CY/3, CY_delta_r/3, CY_delta_ail_lef/3, CY_delta_ail/3
  Product7/1 -> Add4/6
  dlef/1 -> Product6/1, Product4/2, Product/2, Product1/2
  alpha Prelookup/1 -> CY/1, dCY_p_lef/1, CY_p/1, dCY_r_lef/1, CY_r/1, CY_delta_r/1, CY_delta_ail_lef/1, CY_delta_ail/1, CY_lef/1
  Add4/1 -> Cy_tot/1
  Add5/1 -> Product2/1
  CY_p/1 -> Add7/1, Coeff_CY_p/1
  Add1/1 -> Add2/3, Add5/1, [delta_CY_delta_ail]
  CY_lef/1 -> Coeff_CY_lef/1, Add2/2, Add/2
  Add/1 -> Product/1
  dCY_p_lef/1 -> Coeff_dCY_p_lef/1, Product6/2
  CY_delta_r/1 -> Add3/1, Coeff_CY_delta_r/1
  CY_delta_ail_lef/1 -> Coeff_CY_delta_ail_lef/1, Add2/1
  dCY_r_lef/1 -> Coeff_dCY_r_lef/1, Product4/1
  alpha (deg)/1 -> alpha Prelookup/1
  CY_r/1 -> Coeff_CY_r/1, Add6/1
  Product4/1 -> Add6/2
  Add2/1 -> Product1/1
  Product3/1 -> Add4/4
  CY/1 -> Coeff_CY/1, Add3/2, Add1/1, Add/1, Add4/1
  Product2/1 -> Add4/3
  Product/1 -> Add4/2
  alpha Prelookup/2 -> CY/2, CY_p/2, dCY_p_lef/2, dCY_r_lef/2, CY_r/2, CY_delta_r/2, CY_delta_ail_lef/2, CY_delta_ail/2, CY_lef/2
  Product6/1 -> Add7/2
  Add6/1 -> Product5/2
  Add7/1 -> Product7/1
  Product5/1 -> Add4/5
  Product1/1 -> Add5/2
  CY_delta_ail/1 -> Coeff_CY_delta_ail/1, Add1/2
  beta (deg)/1 -> beta Prelookup/1
  Add8/1 -> Gain/1
  drud/1 -> Product3/2
  pb_2v/1 -> Product7/2
  rb_2v/1 -> Product5/1
  right aileron(rad)/1 -> Add8/1
  left aileron(rad)/1 -> Add8/2
  Gain/1 -> Product2/2
  right elevator/1 -> Add9/1
  left elevator/1 -> Add9/2
  [delta_CY_delta_ail] -> Gain2/1
  Add9/1 -> Gain1/1
  Gain1/1 -> Product8/2
  Product8/1 -> Add4/7
  Gain2/1 -> Product8/1

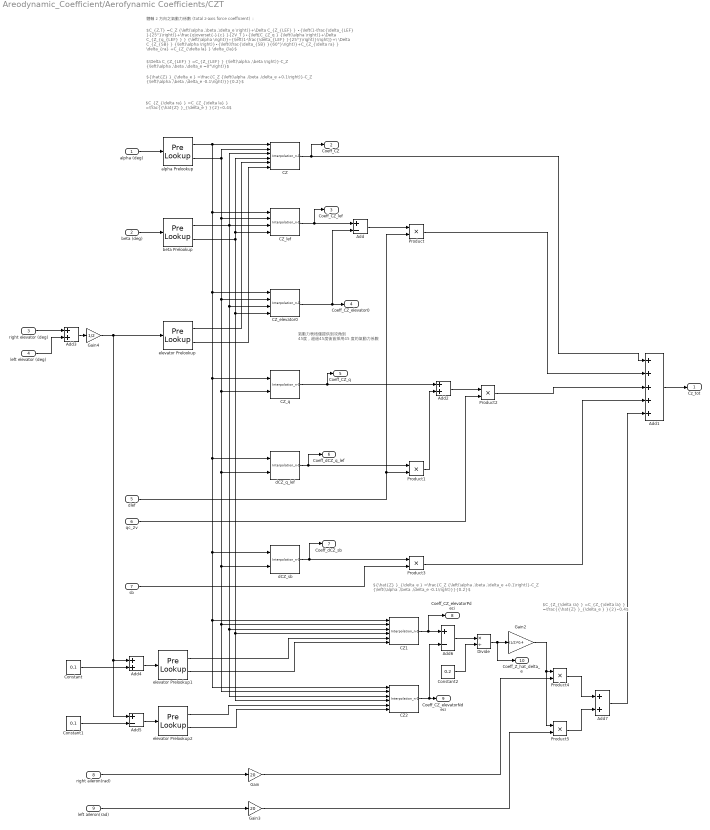
== system Areodynamic_Coefficient/Aerofynamic Coefficients/CZT ==
  note: 氣動力表格僅提供到攻角到
      | 45度，超過45度後皆採用45
      | 度的氣動力係數
  note: ${\hat{Z} }_{\delta_e } =\frac{C_Z {\left(\alpha ,\beta ,\delta_e +0.1\right)}-C_Z {\left(\alpha ,\beta ,\delta_e -0.1\right)}}{0.2}$
  note: $\Delta C_{Z_{LEF} } =C_{Z_{LEF} } {\left(\alpha ,\beta \right)}-C_Z {\left(\alpha ,\beta ,\delta_e =0°\right)}$
  note: $C_{Z,T} =C_Z {\left(\alpha ,\beta ,\delta_e \right)}+\Delta C_{Z_{LEF} } ∙{\left(1-\frac{\delta_{LEF} }{25°}\right)}+\frac{q\overset{-}{c} }{2V_T }∙{\left[C_{Z_q } {\left(\alpha \right)}+\Delta C_{Z_{q_{LEF} } } {\left(\alpha \right)}∙{\left(1-\frac{\delta_{LEF} }{25°}\right)}\right]}+\ \Delta C_{Z_{SB} } {\left(\alpha \right)}∙{\left(\frac{\delta_{SB} }{60°}\right)}+C_{Z_{\delta ra} } \delta_{ra} +C_{Z_{\delta la} } \delta_{la}$
  note: $C_{Z_{\delta ra} } =C_{Z_{\delta la} } =\frac{{\hat{Z} }_{\delta_e } }{2}∙0.4$
  note: 體軸 z 方向之氣動力係數 (total z-axis force coefficient)：
  note: ${\hat{Z} }_{\delta_e } =\frac{C_Z {\left(\alpha ,\beta ,\delta_e +0.1\right)}-C_Z {\left(\alpha ,\beta ,\delta_e -0.1\right)}}{0.2}$
  note: $C_{Z_{\delta ra} } =C_{Z_{\delta la} } =\frac{{\hat{Z} }_{\delta_e } }{2}∙0.4$
  alpha (deg) : Inport
  beta (deg) : Inport  Port=2
  right elevator (deg) : Inport  Port=3
  left elevator (deg) : Inport  Port=4
  dlef : Inport  Port=5
  qc_2v : Inport  Port=6
  sb : Inport  Port=7
  right aileron(rad) : Inport  Port=8
  left aileron(rad) : Inport  Port=9
  Add : Sum  Inputs=+-
  Add1 : Sum  Inputs=+++++
  Add{2..4,7} (4 alike) : Sum
  Add5 : Sum  Inputs=+-
  Add6 : Sum  Inputs=+-
  CZ : Interpolation_n-D  NumberOfTableDimensions=3  Table=AeroCoeff.CZ
      settings: InputPortMap=u0,u1,u2,u3,u4,u5
  CZ1 : Interpolation_n-D  NumberOfTableDimensions=3  Table=AeroCoeff.CZ
      settings: InputPortMap=u0,u1,u2,u3,u4,u5
  CZ2 : Interpolation_n-D  NumberOfTableDimensions=3  Table=AeroCoeff.CZ
      settings: InputPortMap=u0,u1,u2,u3,u4,u5
  CZ_elevator0 : Interpolation_n-D  Table=AeroCoeff.CZ_elevator0
  CZ_lef : Interpolation_n-D  Table=AeroCoeff.CZ_lef
  CZ_q : Interpolation_n-D  NumberOfTableDimensions=1  Table=AeroCoeff.CZ_q
      settings: InputPortMap=u0,u1
  Constant : Constant  Value=0.1
  Constant1 : Constant  Value=0.1
  Constant2 : Constant  Value=0.2
  Divide : Product  Inputs=*/
  Gain : Gain  Gain=20
  Gain2 : Gain  Gain=(1/2)*0.4
  Gain3 : Gain  Gain=20
  Gain4 : Gain  Gain=1/2
  Product{,1..5} (6 alike) : Product
  alpha Prelookup : PreLookup  BreakpointsData=AeroCoeff.alpha_prelookup  IndexSearchMethod=Linear search  BeginIndexSearchUsingPreviousIndexResult=on  DiagnosticForOutOfRangeInput=Warning
  beta Prelookup : PreLookup  BreakpointsData=AeroCoeff.beta_prelookup  IndexSearchMethod=Linear search  BeginIndexSearchUsingPreviousIndexResult=on  DiagnosticForOutOfRangeInput=Warning
  dCZ_q_lef : Interpolation_n-D  NumberOfTableDimensions=1  Table=AeroCoeff.dCZ_q_lef
      settings: InputPortMap=u0,u1
  dCZ_sb : Interpolation_n-D  NumberOfTableDimensions=1  Table=AeroCoeff.dCZ_sb
      settings: InputPortMap=u0,u1
  elevator Prelookup : PreLookup  BreakpointsData=AeroCoeff.elevator_prelookup2  IndexSearchMethod=Linear search  BeginIndexSearchUsingPreviousIndexResult=on  DiagnosticForOutOfRangeInput=Warning
  elevator Prelookup1 : PreLookup  BreakpointsData=AeroCoeff.elevator_prelookup2  IndexSearchMethod=Linear search  BeginIndexSearchUsingPreviousIndexResult=on  DiagnosticForOutOfRangeInput=Warning
  elevator Prelookup2 : PreLookup  BreakpointsData=AeroCoeff.elevator_prelookup2  IndexSearchMethod=Linear search  BeginIndexSearchUsingPreviousIndexResult=on  DiagnosticForOutOfRangeInput=Warning
  Cz_tot : Outport  VectorParamsAs1DForOutWhenUnconnected=off
  Coeff_CZ : Outport  Port=2
  Coeff_CZ_lef : Outport  Port=3
  Coeff_CZ_elevator0 : Outport  Port=4
  Coeff_CZ_q : Outport  Port=5
  Coeff_dCZ_q_lef : Outport  Port=6
  Coeff_dCZ_sb : Outport  Port=7
  Coeff_CZ_elevatorPdeci : Outport  Port=8
  Coeff_CZ_elevatorNdeci : Outport  Port=9
  Coeff_Z_hat_delta_e : Outport  Port=10
  wires:
  Product2/1 -> Add1/3
  alpha Prelookup/2 -> dCZ_q_lef/2, dCZ_sb/2, CZ2/2, CZ1/2, CZ_q/2, CZ_elevator0/2, CZ_lef/2, CZ/2
  Add1/1 -> Cz_tot/1
  elevator Prelookup/1 -> CZ/5
  CZ_q/1 -> Coeff_CZ_q/1, Add2/1
  beta Prelookup/2 -> CZ/4, CZ_lef/4, CZ_elevator0/4, CZ2/4, CZ1/4
  CZ_lef/1 -> Coeff_CZ_lef/1, Add/1
  dCZ_q_lef/1 -> Coeff_dCZ_q_lef/1, Product1/1
  Product1/1 -> Add2/2
  Add2/1 -> Product2/1
  CZ_elevator0/1 -> Add/2, Coeff_CZ_elevator0/1
  Add/1 -> Product/1
  dlef/1 -> Product1/2, Product/2
  Product/1 -> Add1/2
  CZ/1 -> Coeff_CZ/1, Add1/1
  beta Prelookup/1 -> CZ/3, CZ_elevator0/3, CZ2/3, CZ1/3, CZ_lef/3
  alpha Prelookup/1 -> dCZ_q_lef/1, CZ1/1, CZ2/1, dCZ_sb/1, CZ_q/1, CZ_elevator0/1, CZ_lef/1, CZ/1
  alpha (deg)/1 -> alpha Prelookup/1
  elevator Prelookup/2 -> CZ/6
  qc_2v/1 -> Product2/2
  beta (deg)/1 -> beta Prelookup/1
  sb/1 -> Product3/2
  dCZ_sb/1 -> Coeff_dCZ_sb/1, Product3/1
  Product3/1 -> Add1/4
  Constant1/1 -> Add5/2
  CZ2/1 -> Coeff_CZ_elevatorNdeci/1, Add6/2
  Constant/1 -> Add4/2
  Add5/1 -> elevator Prelookup2/1
  Product5/1 -> Add7/2
  Add4/1 -> elevator Prelookup1/1
  left aileron(rad)/1 -> Gain3/1
  Divide/1 -> Coeff_Z_hat_delta_e/1, Gain2/1
  right aileron(rad)/1 -> Gain/1
  Add6/1 -> Divide/1
  Gain2/1 -> Product5/1, Product4/1
  CZ1/1 -> Coeff_CZ_elevatorPdeci/1, Add6/1
  Product4/1 -> Add7/1
  Add3/1 -> Gain4/1
  right elevator (deg)/1 -> Add3/1
  left elevator (deg)/1 -> Add3/2
  elevator Prelookup1/1 -> CZ1/5
  elevator Prelookup1/2 -> CZ1/6
  elevator Prelookup2/1 -> CZ2/5
  elevator Prelookup2/2 -> CZ2/6
  Constant2/1 -> Divide/2
  Add7/1 -> Add1/5
  Gain/1 -> Product4/2
  Gain3/1 -> Product5/2
  Gain4/1 -> elevator Prelookup/1, Add5/1, Add4/1

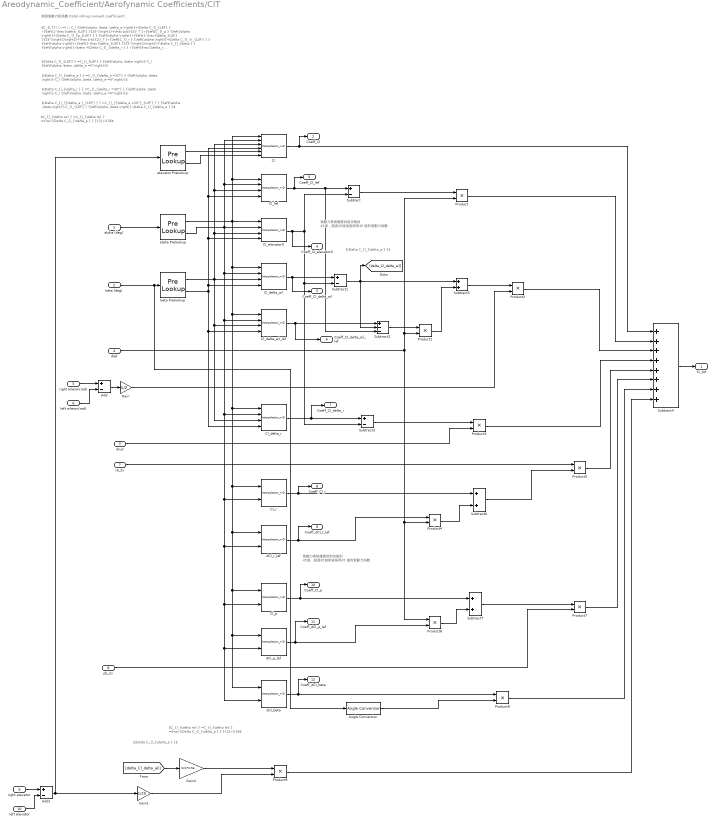
== system Areodynamic_Coefficient/Aerofynamic Coefficients/ClT ==
  note: $\Delta C_{l_{\delta_a } }$
  note: $\Delta C_{l_{{\delta_a }_{LEF} } } =C_{l_{{\delta_a =20°}_{LEF} } } {\left(\alpha ,\beta \right)}-C_{l_{LEF} } {\left(\alpha ,\beta \right)}-\Delta C_{l_{\delta_a } }$
  note: $\Delta C_{l_{\delta_r } } =C_{l_{\delta_r =30°} } {\left(\alpha ,\beta \right)}-C_l {\left(\alpha ,\beta ,\delta_e =0°\right)}$
  note: $\Delta C_{l_{\delta_a } } =C_{l_{\delta_a =20°} } {\left(\alpha ,\beta \right)}-C_l {\left(\alpha ,\beta ,\delta_e =0°\right)}$
  note: $\Delta C_{l_{LEF} } =C_{l_{LEF} } {\left(\alpha ,\beta \right)}-C_l {\left(\alpha ,\beta ,\delta_e =0°\right)}$
  note: 側滾氣動力矩係數 (total rolling moment coefficient)：
  note: 氣動力表格僅提供到攻角到
      | 45度，超過45度後皆採用45
      | 度的氣動力係數
  note: 氣動力表格僅提供到攻角到
      | 45度，超過45度後皆採用45
      | 度的氣動力係數
  note: $C_{l,T} \ \ \ =\ \ \ C_l {\left(\alpha ,\beta ,\delta_e \right)}+\Delta C_{l_{LEF} } ∙{\left(1-\frac{\delta_{LEF} }{25°}\right)}+\frac{pb}{2V_T }∙{\left[C_{l_p } {\left(\alpha \right)}+\Delta C_{l_{p_{LEF} } } {\left(\alpha \right)}∙{\left(1-\frac{\delta_{LEF} }{25°}\right)}\right]}+\frac{rb}{2V_T }∙{\left[C_{l_r } {\left(\alpha \right)}+\Delta C_{l_{r_{LEF} } } {\left(\alpha \right)}∙{\left(1-\frac{\delta_{LEF} }{25°}\right)}\right]}+\Delta C_{l_{\beta } } {\left(\alpha \right)}∙\beta +\Delta C_{l_{\delta_r } } ∙{\left(\frac{\delta_r }{30°}\right)}+\frac{{\left[\Delta C_{l_{\delta_a } } +\Delta C_{l_{{\delta_a }_{LEF} } } ∙{\left(1-\frac{\delta_{LEF} }{25°}\right)}\right]}}{2}∙{\left(\frac{\delta_{ra} }{20°}\right)}-\frac{{\left[\Delta C_{l_{\delta_a } } +\Delta C_{l_{{\delta_a }_{LEF} } } ∙{\left(1-\frac{\delta_{LEF} }{25°}\right)}\right]}}{2}∙{\left(\frac{\delta_{la} }{20°}\right)}+C_{l_{\delta re} } ∙{\left(\frac{\delta_{re} }{25°}\right)}-C_{l_{\delta le} } ∙{\left(\frac{\delta_{le} }{25°}\right)}$
  note: $C_{l_{\delta re} } =C_{l_{\delta le} } =\frac{\Delta C_{l_{\delta_a } } }{2}∙0.56$
  note: $\Delta C_{l_{\delta_a } }$
  note: $C_{l_{\delta re} } =C_{l_{\delta le} } =\frac{\Delta C_{l_{\delta_a } } }{2}∙0.56$
  alpha (deg) : Inport
  beta (deg) : Inport  Port=2
  drud : Inport  Port=3
  dlef : Inport  Port=4
  right aileron(rad) : Inport  Port=5
  left aileron(rad) : Inport  Port=6
  rb_2v : Inport  Port=7
  pb_2v : Inport  Port=8
  right elevator : Inport  Port=9
  left elevator : Inport  Port=10
  Add : Sum  Inputs=+-
  Add1 : Sum  Inputs=+-
  Angle Conversion : aerolibconvert2/Angle Conversion  IU=deg  OU=rad
  Cl : Interpolation_n-D  NumberOfTableDimensions=3  Table=AeroCoeff.Cl
      settings: InputPortMap=u0,u1,u2,u3,u4,u5
  Cl_delta_ail : Interpolation_n-D  Table=AeroCoeff.Cl_delta_ail  InternalRulePriority=Speed
  Cl_delta_ail_lef : Interpolation_n-D  Table=AeroCoeff.Cl_delta_ail_lef  InternalRulePriority=Speed
  Cl_delta_r : Interpolation_n-D  Table=AeroCoeff.Cl_delta_r  InternalRulePriority=Speed
  Cl_elevator0 : Interpolation_n-D  Table=AeroCoeff.Cl_elevator0
  Cl_lef : Interpolation_n-D  Table=AeroCoeff.Cl_lef  InternalRulePriority=Speed
  Cl_p : Interpolation_n-D  NumberOfTableDimensions=1  Table=AeroCoeff.Cl_p  InternalRulePriority=Speed
      settings: InputPortMap=u0,u1
  Cl_r : Interpolation_n-D  NumberOfTableDimensions=1  Table=AeroCoeff.Cl_r  InternalRulePriority=Speed
      settings: InputPortMap=u0,u1
  Gain : Gain  Gain=1/2
  Gain1 : Gain  Gain=1/25
  Gain2 : Gain  Gain=(1/2)*0.56
  Product{,1..9} (10 alike) : Product
  Subtract : Sum  Inputs=+-
  Subtract1 : Sum  Inputs=+-
  Subtract2 : Sum  Inputs=+--
  Subtract3 : Sum  Inputs=+-
  Subtract4 : Sum  Inputs=++++++++
  Subtract5 : Sum
  Subtract6 : Sum
  Subtract7 : Sum
  alpha Prelookup : PreLookup  BreakpointsData=AeroCoeff.alpha_prelookup  IndexSearchMethod=Linear search  BeginIndexSearchUsingPreviousIndexResult=on  DiagnosticForOutOfRangeInput=Warning
  beta Prelookup : PreLookup  BreakpointsData=AeroCoeff.beta_prelookup  IndexSearchMethod=Linear search  BeginIndexSearchUsingPreviousIndexResult=on  DiagnosticForOutOfRangeInput=Warning
  dCl_beta : Interpolation_n-D  NumberOfTableDimensions=1  Table=AeroCoeff.dCl_beta  InternalRulePriority=Speed
      settings: InputPortMap=u0,u1
  dCl_p_lef : Interpolation_n-D  NumberOfTableDimensions=1  Table=AeroCoeff.dCl_p_lef  InternalRulePriority=Speed
      settings: InputPortMap=u0,u1
  dCl_r_lef : Interpolation_n-D  NumberOfTableDimensions=1  Table=AeroCoeff.dCl_r_lef  InternalRulePriority=Speed
      settings: InputPortMap=u0,u1
  elevator Prelookup : PreLookup  BreakpointsData=AeroCoeff.elevator_prelookup1  IndexSearchMethod=Linear search  BeginIndexSearchUsingPreviousIndexResult=on  DiagnosticForOutOfRangeInput=Warning
  Cl_tot : Outport  VectorParamsAs1DForOutWhenUnconnected=off
  Coeff_Cl : Outport  Port=2
  Coeff_Cl_lef : Outport  Port=3
  Coeff_Cl_elevator0 : Outport  Port=4
  Coeff_Cl_delta_ail : Outport  Port=5
  Coeff_Cl_delta_ail_lef : Outport  Port=6
  Coeff_Cl_delta_r : Outport  Port=7
  Coeff_Cl_r : Outport  Port=8
  Coeff_dCl_r_lef : Outport  Port=9
  Coeff_Cl_p : Outport  Port=10
  Coeff_dCl_p_lef : Outport  Port=11
  Coeff_dCl_beta : Outport  Port=12
  wires:
  Cl_elevator0/1 -> Coeff_Cl_elevator0/1, Subtract3/2, Subtract1/2, Subtract/2
  beta Prelookup/1 -> Cl/3, Cl_lef/3, Cl_elevator0/3, Cl_delta_r/3, Cl_delta_ail_lef/3, Cl_delta_ail/3
  Cl_delta_r/1 -> Coeff_Cl_delta_r/1, Subtract3/1
  Cl_lef/1 -> Coeff_Cl_lef/1, Subtract2/3, Subtract/1
  Subtract/1 -> Product/1
  Product6/1 -> Subtract7/2
  alpha Prelookup/1 -> Cl/1, Cl_lef/1, dCl_r_lef/1, dCl_p_lef/1, dCl_beta/1, Cl_p/1, Cl_r/1, Cl_delta_r/1, Cl_delta_ail_lef/1, Cl_delta_ail/1, Cl_elevator0/1
  Product2/1 -> Subtract4/3
  Cl_p/1 -> Coeff_Cl_p/1, Subtract7/1
  beta (deg)/1 -> Angle Conversion/1, beta Prelookup/1
  Subtract2/1 -> Product1/1
  alpha Prelookup/2 -> Cl/2, Cl_lef/2, Cl_r/2, dCl_r_lef/2, dCl_p_lef/2, dCl_beta/2, Cl_p/2, Cl_delta_r/2, Cl_delta_ail_lef/2, Cl_delta_ail/2, Cl_elevator0/2
  alpha (deg)/1 -> alpha Prelookup/1
  Product/1 -> Subtract4/2
  Subtract6/1 -> Product5/2
  rb_2v/1 -> Product5/1
  Cl_delta_ail/1 -> Coeff_Cl_delta_ail/1, Subtract1/1
  Subtract5/1 -> Product2/1
  drud/1 -> Product3/2
  elevator Prelookup/1 -> Cl/5
  Product7/1 -> Subtract4/6
  Subtract7/1 -> Product7/1
  Product5/1 -> Subtract4/5
  dCl_r_lef/1 -> Coeff_dCl_r_lef/1, Product4/1
  Subtract3/1 -> Product3/1
  Subtract1/1 -> Subtract2/2, Subtract5/1, [delta_Cl_delta_ail]
  dlef/1 -> Product6/1, Product4/2, Product/2, Product1/2
  Product3/1 -> Subtract4/4
  Cl_delta_ail_lef/1 -> Coeff_Cl_delta_ail_lef/1, Subtract2/1
  beta Prelookup/2 -> Cl/4, Cl_lef/4, Cl_elevator0/4, Cl_delta_ail/4, Cl_delta_r/4, Cl_delta_ail_lef/4
  Product4/1 -> Subtract6/2
  dCl_beta/1 -> Coeff_dCl_beta/1, Product8/1
  Product1/1 -> Subtract5/2
  dCl_p_lef/1 -> Coeff_dCl_p_lef/1, Product6/2
  Product8/1 -> Subtract4/7
  Cl_r/1 -> Coeff_Cl_r/1, Subtract6/1
  elevator Prelookup/2 -> Cl/6
  Cl/1 -> Coeff_Cl/1, Subtract4/1
  Subtract4/1 -> Cl_tot/1
  pb_2v/1 -> Product7/2
  right aileron(rad)/1 -> Add/1
  left aileron(rad)/1 -> Add/2
  Add/1 -> Gain/1
  Gain/1 -> Product2/2
  right elevator/1 -> Add1/1
  left elevator/1 -> Add1/2
  Add1/1 -> Gain1/1, elevator Prelookup/1
  Gain1/1 -> Product9/2
  [delta_Cl_delta_ail] -> Gain2/1
  Product9/1 -> Subtract4/8
  Gain2/1 -> Product9/1
  Angle Conversion/1 -> Product8/2
